simulink subsystem "storage_TC"  (R2024b)
settings: Solver=VariableStepAuto  StartTime=0.0  StopTime=10.0  RelTol=1e-3
model mask{D=1, H=1.5, n=61, V_var=60, V_min=10, U=5, eps=2, T_amb=20}
  mask prompts: D "Diameter [m]"; H "Height [m]"; n "n (number of volumes - odd integer >= 3)"; V_var "V_var (bottom (V1) + top (Vn)) [%total volume]"; V_min "V_min (V1 and Vn threshold for fixed mesh) [%total volume]"; U "U [W/(K.m2)]"; eps "eps (diffusion/conduction/axial mixing) [W/(K.m)]"; T_amb "T_amb [°C]"
settings Model: Creator=nerotb  LastModifiedBy=nerotb

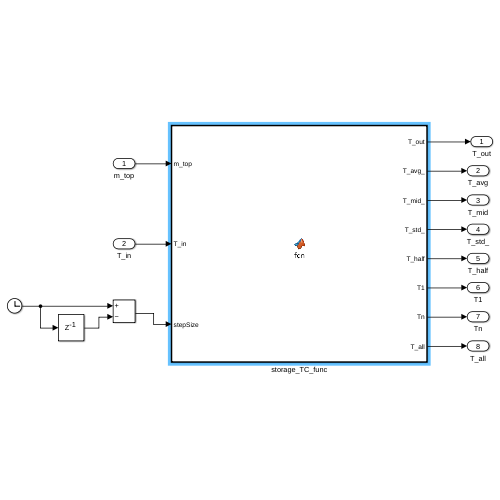
[thumbnail: Simulink's stored preview of the top-level diagram]
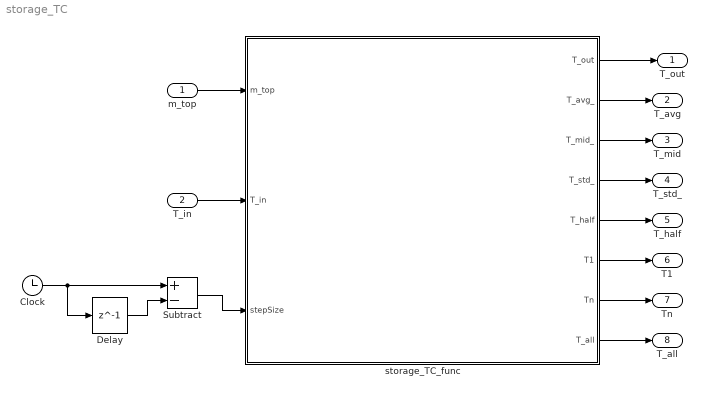
== system storage_TC ==
  m_top : Inport
  T_in : Inport  Port=2
  Clock : Clock
  Delay : Delay  DelayLength=1  InputProcessing=Columns as channels (frame based)
  Subtract : Sum  Inputs=+-
  storage_TC_func : MATLAB Function  TreatAsAtomicUnit=on
  T_out : Outport
  T_avg : Outport  Port=2
  T_mid : Outport  Port=3
  T_std_ : Outport  Port=4
  T_half : Outport  Port=5
  T1 : Outport  Port=6
  Tn : Outport  Port=7
  T_all : Outport  Port=8  PortDimensions=n
  wires:
  storage_TC_func/3(T_mid_) -> T_mid/1
  storage_TC_func/1(T_out) -> T_out/1
  T_in/1 -> storage_TC_func/2(T_in)
  Subtract/1 -> storage_TC_func/3(stepSize)
  m_top/1 -> storage_TC_func/1(m_top)
  storage_TC_func/4(T_std_) -> T_std_/1
  Delay/1 -> Subtract/2
  storage_TC_func/2(T_avg_) -> T_avg/1
  Clock/1 -> Delay/1, Subtract/1
  storage_TC_func/5(T_half) -> T_half/1
  storage_TC_func/6(T1) -> T1/1
  storage_TC_func/7(Tn) -> Tn/1
  storage_TC_func/8(T_all) -> T_all/1

== matlab function storage_TC/storage_TC_func ==
  settings: updateMethod=DISCRETE
  data: m_top input size=1; T_out output size=1; T_in input; stepSize input; H parameter; D parameter; n parameter; V_var parameter; V_min parameter; U parameter; eps parameter; T_amb parameter; T_avg_ output size=1; T_mid_ output size=1; T_std_ output size=1; T_half output size=1; T1 output size=1; Tn output size=1; T_all output [..1000]
function [T_out, T_avg_, T_mid_, T_std_, T_half, T1, Tn, T_all] = fcn(m_top, T_in, stepSize, H, D, n, V_var, V_min, U, eps, T_amb)
%% Description of the model
% This model is a transcription of:
% 
%     [1] K. M. Powell and T. F. Edgar, ‘An adaptive-grid model for dynamic simulation of thermocline thermal energy storage systems’, 
%     Energy Conversion and Management, vol. 76, pp. 865–873, Dec. 2013, doi: 10.1016/j.enconman.2013.08.043.
%
% See 'Implementation constraints' before use.
%
% Main ideas are:
% - 1D vertical mesh
% - meshing is done using n nodes
%     - volumes of node 1 (same for node n) may vary as long as one of the two conditions is respected:
%           - it is larger than a minimal volume
%           - the position of the remaining nodes depicts the thermocline in an accurate way
%       if these conditions are not respected, the tank is operated in a
%       fixed-thermocline mode
%     - other nodes have a constant volume (but their position may vary)
% 
% Main hypothesis:
% - water is incompressible (i.e constant rho)
% - thermal mass capacity is constant (i.e constant Cp)

%% Description of the implementation
% - This function is called at each macro time step
% - When called, a PDE system is solved using ode23. 
% - The solving is done on the time interval (0, dt), where dt is the macro time step 
% - Initial conditions of call at macro time step t+dt are the final
% conditions (solving results) at time step t. 
% Hence the use of persistent variables

%% Input/output variables
% m_top [kg/s]: mass flow entering the tank
% - if m_top > 0:
%     - water enters the tank at the top at temperature T_in and mass flow m_top
%     - same mass flow exits the tank at the bottom at temperature T_out  (note that T_out < T_in is typically verified if temperature stratification occurs)
% - if m_top < 0
%     - water enters the tank at the bottom at temperature T_in and mass flow |m_top|
%     - same mass flow exits the tank at the top at temperature T_out (note that T_in < T_out is typically verified if temperature stratification occurs)
%
% T_avg_ [°C]: average temperature of the tank
% T_mid_ [°C]: temperature of the median node, which may or may not be located at half the height of the tank
% T_half [°C]: temperature of the node which is located at half the height of the tank

%% Implementation constraints
% - The simulation solver must be a fixed time step solver 
%       explanation: this function uses the macro time step as an information for energy balance. 
%       note: first macro time step is supposed to be 30s. Then real macro time
%       step is used.
% - Storage temperatures initializatio:
%       - 20°C (bottom, volume V1)
%       - 55°C (top, volume Vn)
%       - linear variation between V1 and Vn



%% Notes
% - When |m_top| is so large that V1 or Vn would be <0 at the end of the time step, it is cropped
% - epsilon  coefficient is the same for all nodes. 
% Yet, in theory, it should be larger for nodes where thermal stratification (warm fluid above) is not respected. See publication.
% - A too large epislon causes the failure of solving using ode23. A stiff solver would be needed in theses cases

%% Algorithmic complexity
% - There are n+2 variable states: n temperatures and 2 volumes
% - As many equations
% - Complexity can be somehow lowered (or increased) by tuning the 
% tolerance hyperparameters of the solver. Regarding absolute tolerance, be
% careful that volumes are in cubic meters
% - In some cases, increasing the macro time step lowers the complexity only by a small
% extend because the ode solver may anyway chose a fine temporal mesh if
% needed


%% Additional notes
% There seems to exist a mistake in the publication : equation 4C in Table 2



persistent V1
persistent Vn
persistent T_init
persistent T_avg
persistent T_mid
persistent oldStepSize
persistent timeIdx    % index of macro time step. Starts at 1

assert(mod(n, 2));



% dimensions
A = pi * (D ^ 2) / 4 ;                % [m2]
P = pi * D;                           % [m]
V_tot = A * H;                        % [m3]



% discretization
n_TC = n-2;
V_var_ = (V_var /100) * V_tot;  % Volume nodes 1 and n [m3]
V_fixed = V_tot - V_var_;       % volume thermocline zone
V_TC = V_fixed / n_TC;
dx = V_TC / A;                  % [m]
V_min_ = (V_min / 100) * V_tot;





% initialization
if isempty(V1)
    V1 = V_var_/2;
    Vn = V_var_/2;
    T_init = [20, zeros(1, n_TC), 55];
    for idx=1:n_TC
        T_init(idx+1) = 20 + (idx/(n_TC+1)) * (55-20);
    end
    T_mid = T_init(fix(n/2)+1);
    T_avg = T_mid;
    oldStepSize = -1;
    timeIdx = 1;
else
    timeIdx = timeIdx + 1;
end

%% time step check
% - We assume that the current macro time step duration (from p to p+1, `dt` variable) is the same as the previous one (from p-1 to p, `stepSize`)
% - In order to validate this assumption, we check that time step duration
% from p-2 to p-1 (`oldStepSize`) was identical to the one from p-1 to p (`stepSize`)
% (soft check)
% - Here, p is `timeIdx`

if timeIdx == 1                 
    % The passed stepSize value (0) is wrong, let's chose a reasonnable
    % value
    stepSize = 30;
elseif timeIdx == 2
    oldStepSize = stepSize;
else
    assert(abs(oldStepSize- stepSize) < 1e-3) % note: could be done using `isapprox` but `isapprox` is not compatible with C-code generation
end


% temporal parameters
t0 = 0;
tf = stepSize;
dt = tf - t0;

% physical properties
% U          % W / (K.m2) [5, 10]: U = 5   would typically correspond to a full tank discharge in 3 days
% eps        % W / (K.m)  [2,  5]: eps = 2 would typically correspond to an entire temperature homogeneisation (no thermocline) in 3 days
Cp = 4180;   
rho = 1000;
    
    
function out=ODE(t, y, m_top_, m_bottom_, m_down, m_up, T_top, T_bottom)
    % y = [T1, ... , Tn, V1]        n+1 values
    % idx=[1 , ... ,  n, n+1]
    % yp =[T1', ... ,Tn',V1']       n+1 values

    % charge/discharge

    out = zeros(n+1, 1);

    if is_moving_grid
        V1p = (m_bottom_ - m_top_) / rho;               % variation of volume 1
    else
        V1p = 0;
    end

    % node n:
    Vn_ = V_tot - (y(n+1) + (n-2) * V_TC);
    out(n) = (1 / (rho * Cp * Vn_))*...
        ( ...
        - rho*Cp*y(n)*(-V1p) ...
        + Cp * (m_top_*T_top-m_bottom_*y(n)-m_down*y(n)+m_up*y(n-1)) ...
        - U*P*(Vn_/A)*(y(n)-T_amb) ...
        + eps * A * (y(n-1) - y(n)) / dx ...
        );

    % node i: 2 to n-1
    for i=2:n-1
        out(i) = (1 / (rho * Cp * V_TC)) *...
            ( ...
            Cp * (m_up * (y(i-1) - y(i)) + m_down * (y(i+1) - y(i))) ...
            - U * P * dx * (y(i) - T_amb) ...
            + eps * A * (y(i+1) - 2 * y(i) + y(i-1)) / dx ...
            );
    end

    % node 1:
    out(1) = (1 / (rho * Cp * y(n+1)))*...
        ( ...
        - rho*Cp*y(1)*V1p ...
        + Cp * (m_bottom_*T_bottom-m_top_*y(1)+m_down*y(2)-m_up*y(1)) ...
        - U*P*(y(n+1)/A)*(y(1)-T_amb) ...
        + eps * A * (y(2) - y(1)) / dx ...
        );

    out(n+1) = V1p;
end

T_out = 0;
T_avg_ = 0;
T_mid_ = 0;
T_std_ = 0;
T_half = 0;
T1 = 0;
Tn = 0;

loop = true;
while loop
    % eps
    m_top_ = 0;
    m_bottom_ = 0;
    m_up = 0;
    m_down = 0;
    
    
    cond = m_top > 0;      % if true, tank is filled by the top
    condA = (V1 <= V_min_ | T_mid < T_avg);
    condB = (Vn <= V_min_ | T_mid > T_avg);
    
    if cond
        m_top_ = m_top;
        m_bottom_  = 0;
        T_top  = T_in;
        T_bottom   = -10000;  % unused
    
        if condA
            is_moving_grid = false;
            m_down  = m_top_;
            m_up    = 0;
            m_top = 0;
        else
            is_moving_grid = true;
            m_max = V1*rho/dt;
            if m_top_ > m_max
                m_top = m_top_ - 0.99 * m_max;
                fprintf("Storage tank: net flow m_top=%1.2e kg/s is too large for volume V1=%2.2f m3. ", m_top_, V1);
                m_top_ = 0.99 * m_max;     % limit: volume V1 cannot be 0
                fprintf("Storage tank: the function will be called first with %1.2e kg/s and then with %1.2e kg/s.", m_top_, m_top);
            else
                m_top = 0;
            end
            m_down = 0;
            m_up = 0;
        end
    else
        m_top_ = 0;
        m_bottom_  = - m_top;
        T_top = -10000;  % unused
        T_bottom = T_in;
        if condB
            is_moving_grid = false;
            m_down  = 0;
            m_up    = m_bottom_;
            m_top = 0;
        else
            is_moving_grid = true;
            m_max = Vn*rho/dt;
            if m_bottom_ > m_max
                m_top = - (m_bottom_ - 0.99 * m_max);
                fprintf("Storage tank: net flow m_bottom=%1.2e kg/s is too large for volume Vn=%2.2f m3. ", m_bottom_, Vn);
                m_bottom_ = 0.99 * m_max;     % limit: volume Vn cannot be 0
                fprintf("Storage tank: the function will be called first with %1.2e kg/s and then with %1.2e kg/s.", m_bottom_, -m_top);
            else
                m_top = 0;
            end
            m_down = 0;
            m_up = 0;
        end
    end
    
  
    
    
    tspan = [t0, tf];
    options = odeset('RelTol',1e-5, 'AbsTol', 1e-5);
    y0 = [T_init'; V1];
    [~,y] = ode23(@(t, y) ODE(t, y, m_top_, m_bottom_, m_down, m_up, T_top, T_bottom), tspan, y0, options); 
    
    
    
    
    
    %% postprocessing: last time step of ode solving is used to store what will be the initial condition at next call
    % volume
    y_ = zeros(n, 3);
    y_(:, 1) = y(end,1:n)';
    V1 = y(end, n+1);
    Vn = V_tot - (V1 + (n-2) * V_TC);
    
    
    y_(1,2) = V1;
    y_(n,2) = Vn;
    y_(2:n-1,2) = V_TC;
    
    % position
    % note: position is taken at half the height of each volume
    x1 = 0.5 * V1 / A;
    xn = H - 0.5 * Vn / A;
    y_(1,3) = x1;
    y_(n,3) = xn;
    y_(2:n-1,3) = linspace(V1 / A + dx / 2, H - Vn/A - dx/2, n_TC);
    
    % T_avg, T_mid, V1 and T_init
    T_avg = mean(y_(:, 1), Weights=y_(:, 2));
    T_mid = y_(fix(n/2)+1, 1);
    T_init(:) = y_(:, 1);
    T1 = T_init(1);
    Tn = T_init(n);
    
    if cond          % tank is filled by the top
        T_out =  T1; % temperature of node 1 at last time step
    else             % tank is filled by the bottom
        T_out  = Tn; % temperature of node n at last time step
    end
    
    T_avg_ = T_avg;
    T_mid_ = T_mid;
    T_std_ = std(y_(:, 1), y_(:,2));              % weighted standard-deviation
    [~, idx_x_half] = min(abs(y_(:,3)-0.5*H));    % index of the node the closest to half the tank height
    T_half = y_(idx_x_half,1);
    loop = (m_top ~= 0);
end

T_all = T_init';
end
